simulink model "linear_system"  (R2024b)
settings: Solver=FixedStepAuto  StartTime=0.0  StopTime=15  FixedStep=0.01  RelTol=1e-3
undefined symbols (not defined in the file): A_matrix, B_matrix, C_matrix, config, K_lqr, u_trim, x_trim
libraries: simulink x4, uavutilslib x1, uavalgslib x1
settings Model: Creator=kaleb  LastModifiedBy=kaleb

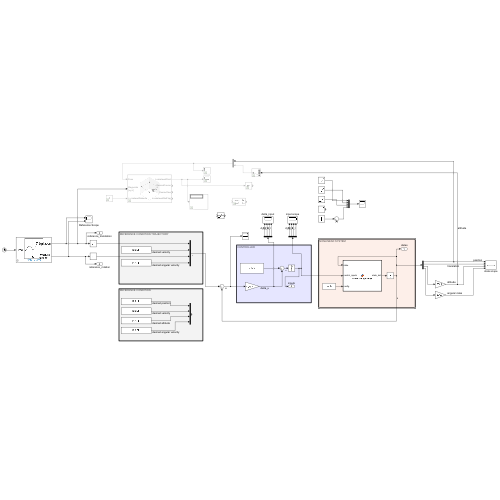
[thumbnail: Simulink's stored preview of the top-level diagram]
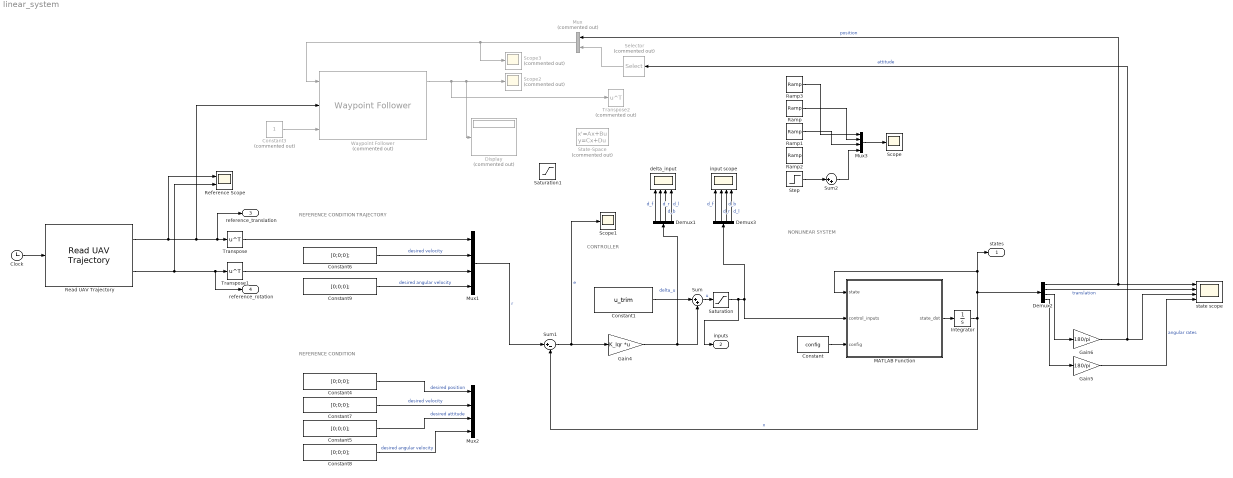
== system linear_system ==
  note: CONTROLLER
  note: REFERENCE CONDITION
  note: NONLINEAR SYSTEM
  note: REFERENCE CONDITION TRAJECTORY
  Clock : Clock
  Constant : Constant  Value=config  OutDataTypeStr=Inherit: Inherit via back propagation
  Constant1 : Constant  Value=u_trim
  Constant3 : Constant  Commented=on
  Constant{4..5,7..9} (5 alike) : Constant  Value=[0;0;0];  SampleTime=-1
  Constant6 : Constant  Value=[0;0;0];  SampleTime=0.1
  Demux1 : Demux
  Demux2 : Demux
  Demux3 : Demux
  Display : Display  Commented=on
  Gain4 : Gain  Gain=K_lqr  Multiplication=Matrix(K*u)
  Gain5 : Gain  Gain=180/pi
  Gain6 : Gain  Gain=180/pi
  Integrator : Integrator  InitialCondition=[x_trim]  ZeroCross=off
  MATLAB Function : MATLAB Function  TreatAsAtomicUnit=on
  Mux : Mux  Commented=on  Inputs=2
  Mux1 : Mux
  Mux2 : Mux
  Mux3 : Mux
  Ramp : simulink/Sources/Ramp  slope=0  start=2  InitialOutput=0.3
  Ramp1 : simulink/Sources/Ramp  slope=0  start=2  InitialOutput=-0.3
  Ramp2 : simulink/Sources/Ramp  slope=-.05  start=0  InitialOutput=-0.3
  Ramp3 : simulink/Sources/Ramp  slope=0  start=2  InitialOutput=0.3
  Read UAV Trajectory : uavutilslib/Read UAV Trajectory  TrajectorySource=From trajectory object in workspace  ScenarioObj=singleUAVScenario  PlatformName=UAV  TrajectoryObj=T  TransformToENU=off  FrameConversionDisplay=NED → NED
  Reference Scope : Scope  NumInputPorts=2
  Saturation : Saturate  UpperLimit=100  LowerLimit=-100
  Saturation1 : Saturate
  Scope : Scope
  Scope1 : Scope
  Scope2 : Scope  Commented=on
  Scope3 : Scope  Commented=on
  Selector : Selector  Commented=on  InputPortWidth=3  IndexOptions=Index vector (dialog)  Indices=[3]  OutputSizes=1
  State-Space : StateSpace  Commented=on  A=double(A_matrix)  B=double(B_matrix)  C=C_matrix  D=zeros(12,4)  InitialCondition=[0 0 0 0 0 0 0 0 0 0 0 0]
  Step : Step  Time=0  Before=-0.3  After=-0.5  SampleTime=0
  Sum : Sum  Inputs=|++
  Sum1 : Sum  Inputs=|+-
  Sum2 : Sum  Inputs=|++
  Transpose : Math  Operator=transpose
  Transpose1 : Math  Operator=transpose
  Transpose2 : Math  Commented=on  Operator=transpose
  Waypoint Follower : uavalgslib/Waypoint Follower  Commented=on  UAVType=multirotor  StartFrom=first  TransitionRadiusSource=internal  TransitionRadius=10  MinLookaheadDistance=0.1  HoverAtLastWaypoint=off  YawInput=off  ShowCrossTrackErrorOutput=off  ShowStatusOutput=off  SimulateUsing=Interpreted execution
  delta_input : Scope  NumInputPorts=4
  input scope : Scope  NumInputPorts=4
  state scope : Scope  NumInputPorts=4
  states : Outport
  inputs : Outport  Port=2
  reference_translation : Outport  Port=3
  reference_rotation : Outport  Port=4
  wires:
  Demux2/1 -> Mux/1, state scope/1  "position"
  Demux2/2 -> state scope/2  "translation"
  Demux2/3 -> Gain6/1
  Demux2/4 -> Gain5/1
  Gain5/1 -> state scope/4  "angular rates"
  Gain6/1 -> Selector/1, state scope/3  "attitude"
  Constant9/1 -> Mux1/4  "desired angular velocity"
  Constant6/1 -> Mux1/2  "desired velocity"
  Clock/1 -> Read UAV Trajectory/1
  Read UAV Trajectory/2 -> reference_rotation/1, Transpose1/1, Reference Scope/2
  Demux3/3 -> input scope/3  "d_b"
  Demux3/1 -> input scope/1  "d_f"
  MATLAB Function/1(state_dot) -> Integrator/1
  Sum1/1 -> Scope1/1, Gain4/1  "e"
  Demux3/2 -> input scope/2  "d_r"
  Integrator/1 -> Demux2/1, states/1, MATLAB Function/1(state), Sum1/2  "x"
  Demux3/4 -> input scope/4  "d_l"
  Constant1/1 -> Sum/1
  Gain4/1 -> Sum/2, Demux1/1  "delta_u"
  Demux1/2 -> delta_input/2  "d_r"
  Demux1/1 -> delta_input/1  "d_f"
  Demux1/3 -> delta_input/3  "d_b"
  Demux1/4 -> delta_input/4  "d_l"
  Constant5/1 -> Mux2/3  "desired attitude"
  Constant7/1 -> Mux2/2  "desired velocity"
  Constant8/1 -> Mux2/4  "desired angular velocity"
  Constant4/1 -> Mux2/1  "desired position"
  Transpose1/1 -> Mux1/3
  Transpose/1 -> Mux1/1
  Selector/1 -> Mux/2
  Mux/1 -> Scope3/1, Waypoint Follower/1
  Ramp3/1 -> Mux3/1
  Ramp/1 -> Mux3/2
  Ramp1/1 -> Mux3/3
  Mux3/1 -> Scope/1
  Sum/1 -> Saturation/1  "u"
  Saturation/1 -> inputs/1, Demux3/1, MATLAB Function/2(control_inputs)
  Read UAV Trajectory/1 -> Waypoint Follower/2, reference_translation/1, Transpose/1, Reference Scope/1
  Constant3/1 -> Waypoint Follower/3
  Waypoint Follower/1 -> Transpose2/1, Display/1, Scope2/1
  Step/1 -> Sum2/1
  Sum2/1 -> Mux3/4
  Mux1/1 -> Sum1/1  "r"
  Constant/1 -> MATLAB Function/3(config)

== matlab function linear_system/MATLAB Function ==
  data: state input; control_inputs input; config input; state_dot output
%% Equation of motion calculation
function state_dot = nonlinear_dynamics(state, control_inputs, config)
t_motor = 31/1000;   % Motor thickness (m)
t_prop = 2/1000;    % Propeller thickness (m)
d_cube = 0.10;    % Cube dimension (m)
m_motor = 100/1000;   % Motor mass (kg)
m_prop = 21/1000;    % Propeller mass (kg)
m_arm = 65/1000;     % Arm mass (kg)
m_cube = 1.74;    % Cube mass (kg)
r_motor = 28/1000;   % Motor radius (m)
r_prop = 25.4/100;    % Propeller radius (m)

g = 9.81; % Gravity (kg/m^2)
k1 = 1;   % Thrust coefficient
k2 = 0.2; % Torque coefficient

[CG_matrix, J_matrix_body, m_tot] = calculate_CG_Moment_of_inertia(config);
X_cg = CG_matrix(1);
Y_cg = CG_matrix(2);

l_f = config(1);
l_r = config(2);
l_b = config(3);
l_l = config(4);

% Extract state variables
pn = state(1); pe = state(2); h = state(3);
u = state(4); v = state(5); w = state(6);
phi = state(7); theta = state(8); psi = state(9);
p = state(10); q = state(11); r = state(12);

% Extract control inputs
delta_f = control_inputs(1);
delta_r = control_inputs(2);
delta_b = control_inputs(3);
delta_l = control_inputs(4);

% Position Dynamics
    position_matrix = [
        cos(theta)*cos(psi), sin(phi)*sin(theta)*cos(psi) - cos(phi)*sin(psi), cos(phi)*sin(theta)*cos(psi) + sin(phi)*sin(psi);
        cos(theta)*sin(psi), sin(phi)*sin(theta)*sin(psi) + cos(phi)*cos(psi), cos(phi)*sin(theta)*sin(psi) - sin(phi)*cos(psi);
        sin(theta), -sin(phi)*cos(theta), -cos(phi)*cos(theta)
    ];
    position_vector = [u; v; w];
    position_dot = position_matrix * position_vector;
    
    % Linear Velocity Dynamics
    linear_velocity_matrix = [
        0, r, -q;
        -r, 0, p;
        q, -p, 0
    ];
    gravity_vector = [-g*sin(theta); g*cos(theta)*sin(phi); g*cos(theta)*cos(phi)];
    control_force = [0; 0; -k1 * (delta_f + delta_r + delta_b + delta_l) / m_tot];
    linear_velocity_dot = linear_velocity_matrix * [u; v; w] + gravity_vector + control_force;
    
    % Angular Velocity Dynamics
    angular_velocity_matrix = [
        1, sin(phi)*tan(theta), cos(phi)*tan(theta);
        0, cos(phi), -sin(phi);
        0, sin(phi)/cos(theta), cos(phi)/cos(theta)
    ];
    angular_velocity_dot = angular_velocity_matrix * [p; q; r];
    
    % Rotational Dynamics
    % Torques due to rotor thrusts
    tau_x = - (l_r-Y_cg) * k1 * delta_r - (l_l-Y_cg) * k1 * delta_l; % Front-back torques
    tau_y = (l_f-X_cg) * k1 * delta_f + (l_b-X_cg) * k1 * delta_b; % Right-left torques
    tau_z = k2 * (-delta_f + delta_r - delta_b + delta_l); % Yaw torque due to rotor drag
    
    % Total torques
    control_torque = [tau_x; tau_y; tau_z];
    
    % Gyroscopic effects
    rotational_dynamics_matrix = [
        (J_matrix_body(2, 2) - J_matrix_body(3, 3)) / J_matrix_body(1, 1), 0, 0;
        0, (J_matrix_body(3, 3) - J_matrix_body(1, 1)) / J_matrix_body(2, 2), 0;
        0, 0, (J_matrix_body(1, 1) - J_matrix_body(2, 2)) / J_matrix_body(3, 3)
    ];
    % rotational_coupling = [q * r; p * r; p * q];
    rotational_coupling = [q * r; p * r; p * q];
    rotational_velocity_dot = rotational_dynamics_matrix * rotational_coupling + (J_matrix_body \ control_torque);
    % rotational_velocity_dot = inv(J_matrix_body) * (control_torque - cross([p;q;r], J_matrix_body*[p;q;r]));
    % Combine EOMs
    
    % Combine EOMs
    state_dot = [position_dot; linear_velocity_dot; angular_velocity_dot; rotational_velocity_dot];
end
